simulink model "mfc_z"  (R2026a)
settings: Solver=VariableStepAuto
InitFcn:
  | guidance_v_ref_omega = deg2rad(100) / (2*pi);   % natural frequency [Hz] = 0.2778 Hz
  | guidance_v_ref_zeta  = 0.85;                     % damping ratio [-]
  | FFilter_T      = 5;
  | WFilter_T      = 50;
  | alpha_T        = 5/airframe.m;
  | kp_T           = 2;
  | kd_T           = 1.5;
  | Umax_T         = (9.81 * airframe.m);
  | Umin_T         = -40;
undefined symbols (not defined in the file): airframe, g, tau_m, Ts
libraries: simulink x3, mfc_lib x1, eeGeneralControl x1, eeStairGenerator x1
settings Model: Creator=devinbellll  LastModifiedBy=devinbellll

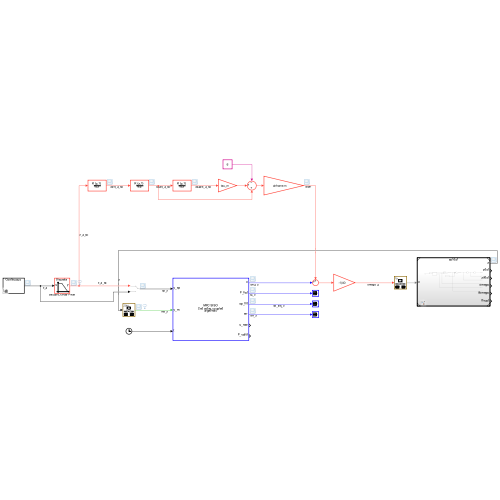
[thumbnail: Simulink's stored preview of the top-level diagram]
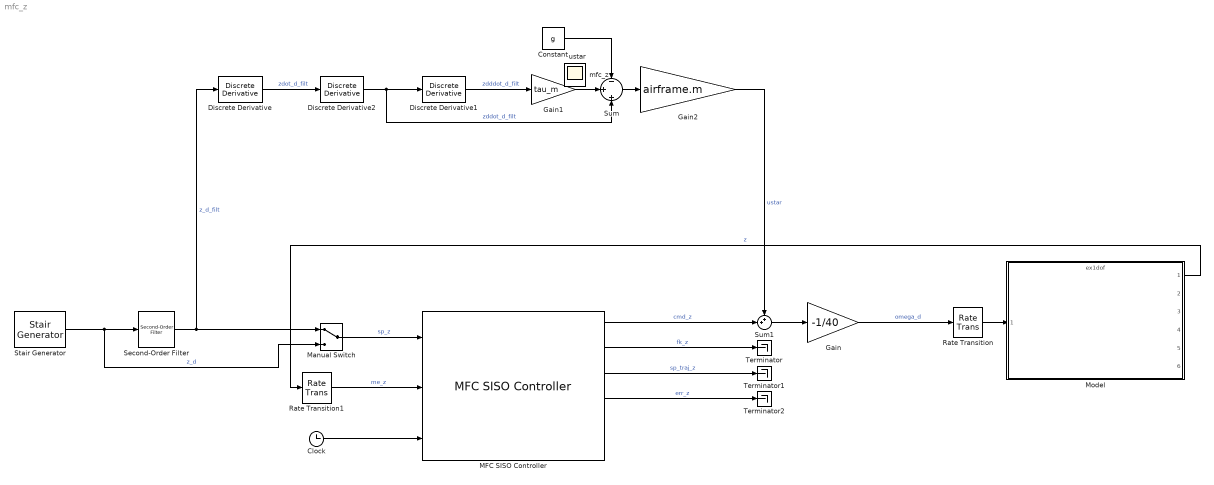
== system mfc_z ==
  Clock : Clock
  Constant : Constant  Value=g
  Discrete Derivative : simulink/Discrete/Discrete Derivative  gainval=1.0  ICPrevScaledInput=0.0  OutMin=[]  OutMax=[]  OutDataType=fixdt(1, 16)  OutScaling=2^-10  DoSatur=off
  Discrete Derivative1 : simulink/Discrete/Discrete Derivative  gainval=1.0  ICPrevScaledInput=0.0  OutMin=[]  OutMax=[]  OutDataType=fixdt(1, 16)  OutScaling=2^-10  DoSatur=off
  Discrete Derivative2 : simulink/Discrete/Discrete Derivative  gainval=1.0  ICPrevScaledInput=0.0  OutMin=[]  OutMax=[]  OutDataType=fixdt(1, 16)  OutScaling=2^-10  DoSatur=off
  Gain : Gain  Gain=-1/40
  Gain1 : Gain  Gain=tau_m
  Gain2 : Gain  Gain=airframe.m
  MFC SISO Controller : mfc_lib/MFC SISO Controller  model_order=Second order (ddot_y = F + alpha*u)  controller_structure=Coupled (error-driven estimator, poles folded)  estimator_type=Algebraic (growing window)  alpha=1/airframe.m  Kp=kp_T^2  Kd=2*kd_T*kp_T  Ki=0  SimulateUsing=Code generation  ref_filter_window=WFilter_T  est_filter_window=FFilter_T  command_filter=1  est_hold_time=0  use_ref_filter=off  use_control_sat=off  u_min=Umin_T  u_max=Umax_T  use_external_command=off  use_live_alpha=off  Ts=0.01
  Manual Switch : ManualSwitch
  Model : ModelReference  ModelNameDialog=ex1dof.slx  SimulationMode=Normal  ModelReferenceVersion=1.17
  Rate Transition : RateTransition
  Rate Transition1 : RateTransition  OutPortSampleTime=1/500
  Second-Order Filter : eeGeneralControl/Second-Order Filter  FilterType=Low-pass  fn=guidance_v_ref_omega  Zeta=guidance_v_ref_zeta  Ts=Ts  A0=0  Ph0=0  f0=0  b0=0
      settings: LibrarySourceBlock=ee_sl_lib/General Control/Second-Order Filter
  Stair Generator : eeStairGenerator/Stair Generator  LabelModeActiveChoice=Continuous  TimeInput=[5]  AmplitudeInput=[-1]  SampleTime=0  RepeatPattern=off  OutDataTypeStr=double
      settings: LibrarySourceBlock=ee_sl_lib/General Control/Stair Generator
  Sum : Sum  Inputs=-|+|+
  Sum1 : Sum  Inputs=++|
  Terminator : Terminator
  Terminator1 : Terminator
  Terminator2 : Terminator
  mfc_z : Scope
      settings: ActiveDisplayYMinimum=-1.1367405205425474  ActiveDisplayYMaximum=0.16746039433152027
  ustar : Scope
      settings: ActiveDisplayYMinimum=-55.584229279158023  ActiveDisplayYMaximum=-2.0895855284930533
  wires:
  Clock/1 -> MFC SISO Controller/3
  Manual Switch/1 -> MFC SISO Controller/1  "sp_z"
  Model/1 -> Rate Transition1/1  "z"
  Stair Generator/1 -> Manual Switch/2, Second-Order Filter/1  "z_d"
  Rate Transition/1 -> Model/1
  Rate Transition1/1 -> MFC SISO Controller/2  "me_z"
  Gain/1 -> Rate Transition/1  "omega_d"
  MFC SISO Controller/2 -> Terminator/1  "fk_z"
  MFC SISO Controller/3 -> Terminator1/1  "sp_traj_z"
  MFC SISO Controller/4 -> Terminator2/1  "err_z"
  Second-Order Filter/1 -> Discrete Derivative/1, Manual Switch/1  "z_d_filt"
  Sum/1 -> Gain2/1
  Gain2/1 -> Sum1/1  "ustar"
  MFC SISO Controller/1 -> Sum1/2  "cmd_z"
  Sum1/1 -> Gain/1
  Discrete Derivative/1 -> Discrete Derivative2/1  "zdot_d_filt"
  Discrete Derivative2/1 -> Sum/3, Discrete Derivative1/1  "zddot_d_filt"
  Discrete Derivative1/1 -> Gain1/1  "zdddot_d_filt"
  Gain1/1 -> Sum/2
  Constant/1 -> Sum/1
